simulink model "untitled1"  (R2015b)
settings: Solver=FixedStepAuto  StartTime=0.0  StopTime=1e-5  RelTol=1e-3
libraries: dsparch4 x1, rfmathmodels1 x1, rfprivate1 x1
settings Model: Creator=dimple  LastModifiedBy=dimple

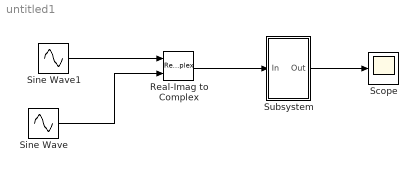
== system untitled1 ==
  Real-Imag to Complex : RealImagToComplex
  Scope : Scope
  Sine Wave : Sin  Frequency=1e6  SampleTime=0
  Sine Wave1 : Sin  Frequency=1e6  Phase=pi/2  SampleTime=0
  Subsystem : Subsystem
  wires:
  Real-Imag to Complex/1 -> Subsystem/1(In)
  Subsystem/1(Out) -> Scope/1
  Sine Wave1/1 -> Real-Imag to Complex/1
  Sine Wave/1 -> Real-Imag to Complex/2

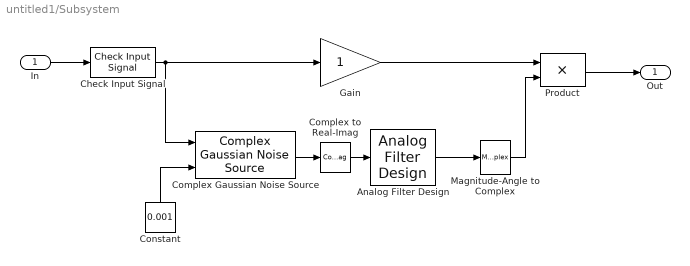
== system untitled1/Subsystem ==
  In : Inport
  Analog Filter Design : dsparch4/Analog Filter Design  method=Butterworth  filttype=Lowpass  N=5  Wlo=1e7  Whi=80  Rp=2  Rs=40
  Check Input Signal : rfmathmodels1/Mixer/Check Input Signal  SystemSampleTime=-1
  Complex Gaussian Noise Source : rfprivate1/Complex Gaussian Noise Source  myseed=2137
  Complex to Real-Imag : ComplexToRealImag  Output=Real
  Constant : Constant  Value=0.001  SampleTime=Inf
  Gain : Gain  SaturateOnIntegerOverflow=on  OutDataTypeStr=Inherit: Same as input  ParamDataTypeStr=Inherit: Same as input
  Magnitude-Angle to Complex : MagnitudeAngleToComplex  Input=Angle  ConstantPart=1
  Product : Product  SaturateOnIntegerOverflow=on  InputSameDT=on  OutDataTypeStr=Inherit: Same as first input
  Out : Outport
  wires:
  Constant/1 -> Complex Gaussian Noise Source/2
  Complex Gaussian Noise Source/1 -> Complex to Real-Imag/1
  Gain/1 -> Product/1
  Check Input Signal/1 -> Complex Gaussian Noise Source/1, Gain/1
  In/1 -> Check Input Signal/1
  Product/1 -> Out/1
  Complex to Real-Imag/1 -> Analog Filter Design/1
  Magnitude-Angle to Complex/1 -> Product/2
  Analog Filter Design/1 -> Magnitude-Angle to Complex/1
